simulink model "Ejercicio14_16_02_17"  (R2013a)
settings: Solver=ode45  StartTime=0.0  StopTime=100  RelTol=1e-3
settings Model: Creator=Miguel  LastModifiedBy=Miguel

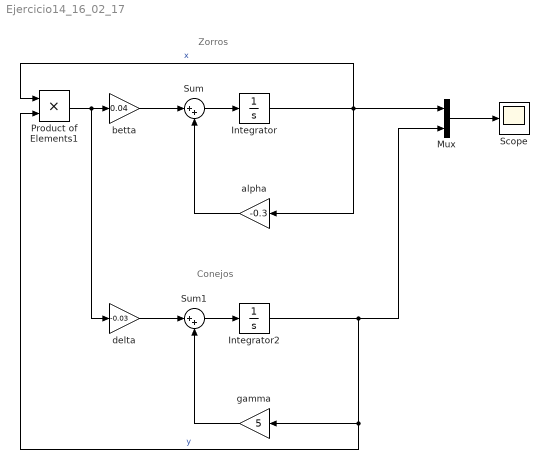
== system Ejercicio14_16_02_17 ==
  note: Conejos
  note: Zorros
  Integrator : Integrator  InitialCondition=3
  Integrator2 : Integrator  InitialCondition=100
  Mux : Mux  Inputs=2
  Product of Elements1 : Product
  Scope : Scope
      settings: ShowLegends=on  TimeRange=10
  Sum : Sum  Inputs=|++
  Sum1 : Sum  Inputs=|++
  alpha : Gain  Gain=-0.3
  betta : Gain  Gain=0.04
  delta : Gain  Gain=-0.03
  gamma : Gain  Gain=5
  wires:
  Sum/1 -> Integrator/1
  Mux/1 -> Scope/1
  alpha/1 -> Sum/2
  Integrator/1 -> alpha/1, Product of Elements1/1, Mux/1  "x"
  Sum1/1 -> Integrator2/1
  gamma/1 -> Sum1/2
  delta/1 -> Sum1/1
  betta/1 -> Sum/1
  Integrator2/1 -> Product of Elements1/2, gamma/1, Mux/2  "y"
  Product of Elements1/1 -> delta/1, betta/1
